simulink model "sl_driveline"  (R2017b)
settings: Solver=ode45  StartTime=0.0  StopTime=10.0  RelTol=1e-3  EnableMultiTasking=on
undefined symbols (not defined in the file): L
libraries: roblocks x2, simulink x1
settings Model: Creator=pic  LastModifiedBy=corkep
settings SolverCC: ZeroCrossAlgorithm=Adaptive
settings DataIOCC: SaveFormat=Array  ReturnWorkspaceOutputs=on  TimeSaveName=t  OutputSaveName=y
settings OptimizationCC: ExpressionDepthLimit=2147483647  LifeSpan=inf
settings DebuggingCC: UnderspecifiedInitializationDetection=Classic  MergeDetectMultiDrivingBlocksExec=none  SolverPrmCheckMsg=warning  AllowSymbolicDim=off  StateNameClashWarn=warning  StrictBusMsg=Warning  SFUnexpectedBacktrackingDiag=warning  SFNoUnconditionalDefaultTransitionDiag=warning  SFExecutionAtInitializationDiag=none
settings HardwareCC: ProdBitPerPointer=32  ProdBitPerSizeT=32  ProdBitPerPtrDiffT=32  ProdLargestAtomicFloat=None  ProdIntDivRoundTo=Undefined  ProdEndianess=Unspecified  ProdWordSize=32  ProdHWDeviceType=32-bit Generic
settings ModelReferenceCC: PropagateSignalLabelsOutOfModel=off
settings CodeAppCC: StateflowObjectComments=on
settings GRTTargetCC: TargetLangStandard=C89/C90 (ANSI)  GeneratePreprocessorConditionals=Disable all  CombineOutputUpdateFcns=off  GRTInterface=on
settings ConfigComp: CovMetricSettings=dw  CovHtmlReporting=on  CovSaveCumulativeToWorkspaceVar=on  CovSaveSingleToWorkspaceVar=on  CovExternalEMLEnable=off

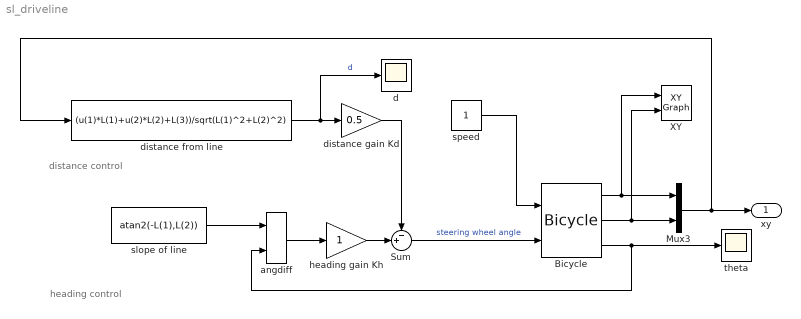
== system sl_driveline ==
  note: distance control
  note: heading control
  Bicycle : roblocks/Vehicles/Bicycle  vlim=1  accel=1  alim=1  steer_rate=Inf  L=1  x0=x0
  Mux3 : Mux  Inputs=2
  Sum : Sum  Inputs=-+|
  XY : simulink/Sinks/XY Graph  xmin=0  xmax=10  ymin=0  ymax=10  st=-1
  angdiff : roblocks/Toolbox/angdiff
  d : Scope
  distance from line : Fcn  Expr=(u(1)*L(1)+u(2)*L(2)+L(3))/sqrt(L(1)^2+L(2)^2)
  distance gain Kd : Gain  Gain=0.5
  heading gain Kh : Gain
  slope of line : Constant  Value=atan2(-L(1),L(2))
  speed : Constant  VectorParams1D=off  SampleTime=0.02
  theta : Scope
  xy : Outport
  wires:
  Mux3/1 -> distance from line/1, xy/1
  slope of line/1 -> angdiff/1
  angdiff/1 -> heading gain Kh/1
  heading gain Kh/1 -> Sum/2
  speed/1 -> Bicycle/1
  Sum/1 -> Bicycle/2  "steering wheel angle"
  distance from line/1 -> distance gain Kd/1, d/1  "d"
  Bicycle/1 -> XY/1, Mux3/1
  Bicycle/2 -> XY/2, Mux3/2
  Bicycle/3 -> angdiff/2, theta/1
  distance gain Kd/1 -> Sum/1
